simulink model "es2_1_cardinal"  (R2024b)
settings: Solver=VariableStepAuto  StartTime=0.0  StopTime=30  RelTol=1e-3
libraries: vrlib x1
settings Model: Creator=danie  LastModifiedBy=danie

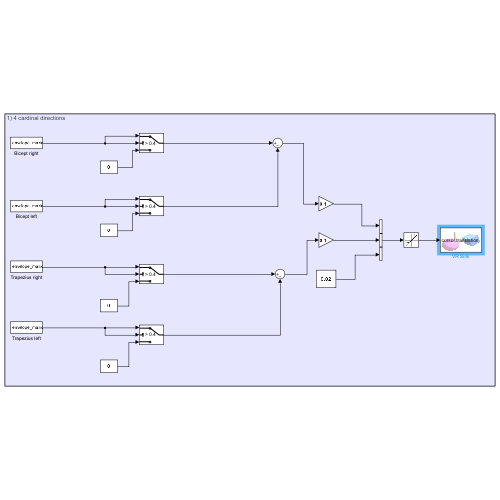
[thumbnail: Simulink's stored preview of the top-level diagram]
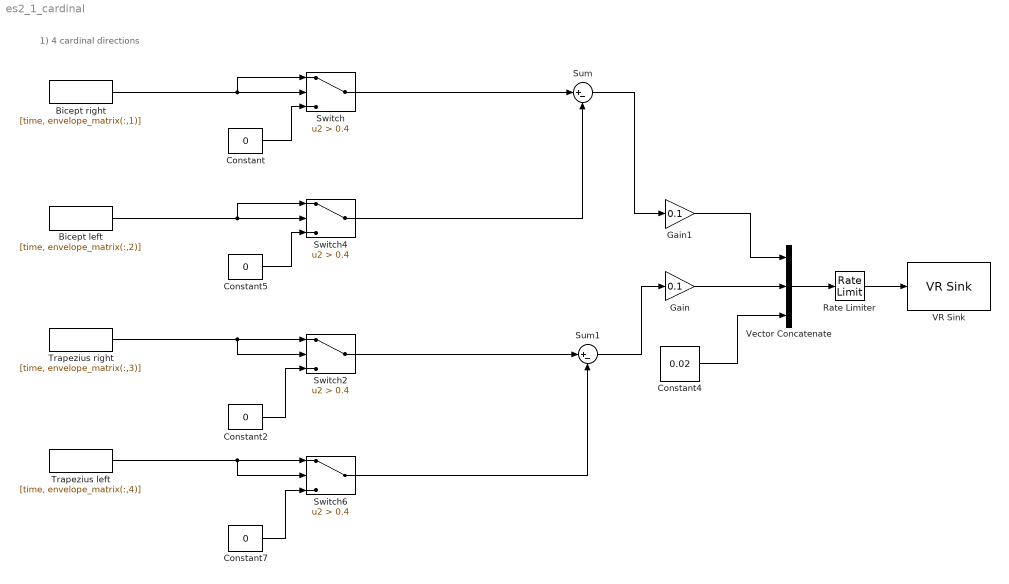
== system es2_1_cardinal ==
  note: 1) 4 cardinal directions
  Bicept left : FromWorkspace  VariableName=[time, envelope_matrix(:,2)]
  Bicept right : FromWorkspace  VariableName=[time, envelope_matrix(:,1)]
  Constant{,2,5,7} (4 alike) : Constant  Value=0
  Constant4 : Constant  Value=0.02
  Gain : Gain  Gain=0.1
  Gain1 : Gain  Gain=0.1
  Rate Limiter : RateLimiter  RisingSlewLimit=0.4  FallingSlewLimit=-0.4  SampleTimeMode=inherited
  Sum : Sum  Inputs=|+-
  Sum1 : Sum  Inputs=|+-
  Switch{,2,4,6} (4 alike) : Switch  Criteria=u2 > Threshold  Threshold=0.4  SaturateOnIntegerOverflow=off  InputSameDT=off
  Trapezius left : FromWorkspace  VariableName=[time, envelope_matrix(:,4)]
  Trapezius right : FromWorkspace  VariableName=[time, envelope_matrix(:,3)]
  VR Sink : vrlib/VR Sink  InstantiateOnLoad=on  SampleTime=0.1  ViewEnable=on  RemoteChange=off  RemoteView=off  FieldsWritten=cursor.translation.3.1.1.double  WorldFileName=8_palline_color.wrl  AutoView=off  VideoDimensions=[]  AllowVariableSize=off
  Vector Concatenate : Concatenate  NumInputs=3
  wires:
  Switch/1 -> Sum/1
  Switch2/1 -> Sum1/1
  Switch6/1 -> Sum1/2
  Constant7/1 -> Switch6/3
  Bicept left/1 -> Switch4/1, Switch4/2
  Constant4/1 -> Vector Concatenate/3
  Constant2/1 -> Switch2/3
  Sum/1 -> Gain1/1
  Switch4/1 -> Sum/2
  Constant/1 -> Switch/3
  Trapezius left/1 -> Switch6/1, Switch6/2
  Vector Concatenate/1 -> Rate Limiter/1
  Sum1/1 -> Gain/1
  Rate Limiter/1 -> VR Sink/1
  Trapezius right/1 -> Switch2/1, Switch2/2
  Constant5/1 -> Switch4/3
  Bicept right/1 -> Switch/2, Switch/1
  Gain1/1 -> Vector Concatenate/1
  Gain/1 -> Vector Concatenate/2
